simulink model "target"  (R2024b)
settings: Solver=FixedStepDiscrete  StartTime=0.0  StopTime=Inf  FixedStep=0.01  MaxStep=1e-5  RelTol=1e-4  EnableMultiTasking=on
InitFcn:
  | Motor_data_IM_R;
undefined symbols (not defined in the file): DiscIntNeverNeededParam, Down, GPTRIP1SEL, imr_min, j, K_r, K_s, ki, Ki_flux, Ki_w, kp, Kp_flux, Kp_w, lim, p, Tau_r, Ts, TZ1, Up, V_dc, wr_n
libraries: c2802xlib x6, slpidlib x2, c2000lib x1, c280xlib x1
settings Model: ExtModeTrigDuration=8  Creator=dario  LastModifiedBy=dario
settings OptimizationCC: DefaultParameterBehavior=Inlined  DefaultUnderspecifiedDataType=single  EnhancedBackFolding=on  PassReuseOutputArgsAs=Individual arguments  MaxStackSize=1024  OptimizeBlockOrder=speed  DifferentSizesBufferReuse=on  OptimizationCustomize=off  EfficientTunableParamExpr=on
settings DebuggingCC: ParameterTunabilityLossMsg=error
settings HardwareCC: ProdBitPerChar=16  ProdBitPerInt=16  ProdBitPerPointer=32  ProdBitPerSizeT=32  ProdBitPerPtrDiffT=32  ProdLargestAtomicInteger=Integer  ProdLargestAtomicFloat=None  ProdWordSize=16  ProdLongLongMode=on  ProdHWDeviceType=Texas Instruments->C2000  HardwareBoardFeatureSet=SoCBlockset
settings SFSimCC: MATLABDynamicMemAlloc=off
settings RTWCC: Description=Embedded Coder  SystemTargetFile=ert.tlc  HardwareBoard=TI Delfino F28379D LaunchPad  TemplateMakefile=ert_default_tmf  GenerateReport=on  Toolchain=Texas Instruments Code Composer Studio (C2000)  LaunchReport=on  CodeProfilingSaveOptions=MetricsOnly
settings CodeAppCC: ForceParamTrailComments=on  IgnoreCustomStorageClasses=off  OperatorAnnotations=on  SimulinkDataObjDesc=on  SFDataObjDesc=on  InsertBlockDesc=on
settings ERTTargetCC: CodeReplacementLibrary=TI C28x  ExtModeTransport=4  ExtModeStaticAlloc=on  ExtModeAutomaticAllocSize=off  ExtModeStaticAllocSize=10000  ExtModeMexFile=ext_xcp  ExtModeIntrfLevel=Level2 - Open

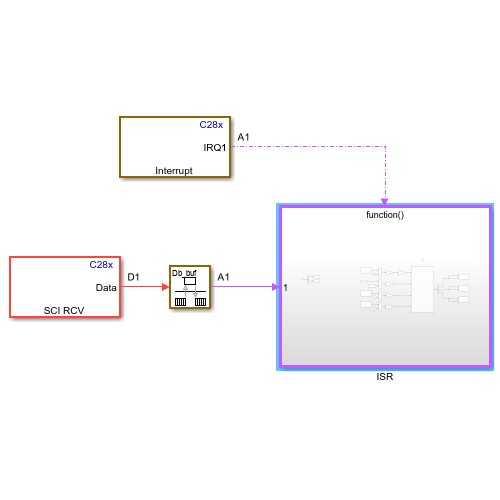
[thumbnail: Simulink's stored preview of the top-level diagram]
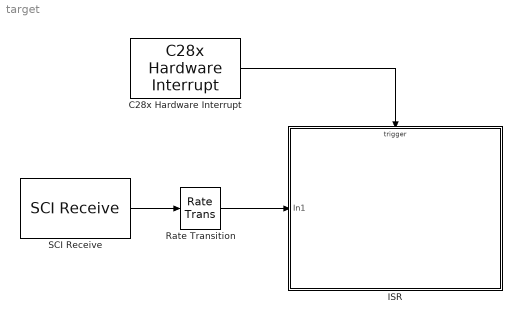
== system target ==
  C28x Hardware Interrupt : c2000lib/Scheduling/C28x Hardware Interrupt  irqnumbers=[1]  pienumbers=[3]  irqpriorities=[30]  irqpreempts=[0]  showinput=off  dspchiptype=C280X
  ISR : Subsystem
  Rate Transition : RateTransition  Deterministic=off
  SCI Receive : c280xlib/SCI Receive  Priority=2  sciModule=A  dataHead='SS'  headerCheckMaxCount=16  dataTail='EE'  dataType=uint16  dataLenOptions=Length via dialog  dataDim=2  maxDataLength=1  initValue=0  errOption=Output the last received value  errValue=0  sampleTime=0.01  blockingMode=off  timeOut=inf  outputStatus=off
      settings: LibrarySourceBlock=c2837xDlib/SCI Receive
  wires:
  C28x Hardware Interrupt/1 -> ISR/Trigger
  Rate Transition/1 -> ISR/1(In1)
  SCI Receive/1 -> Rate Transition/1

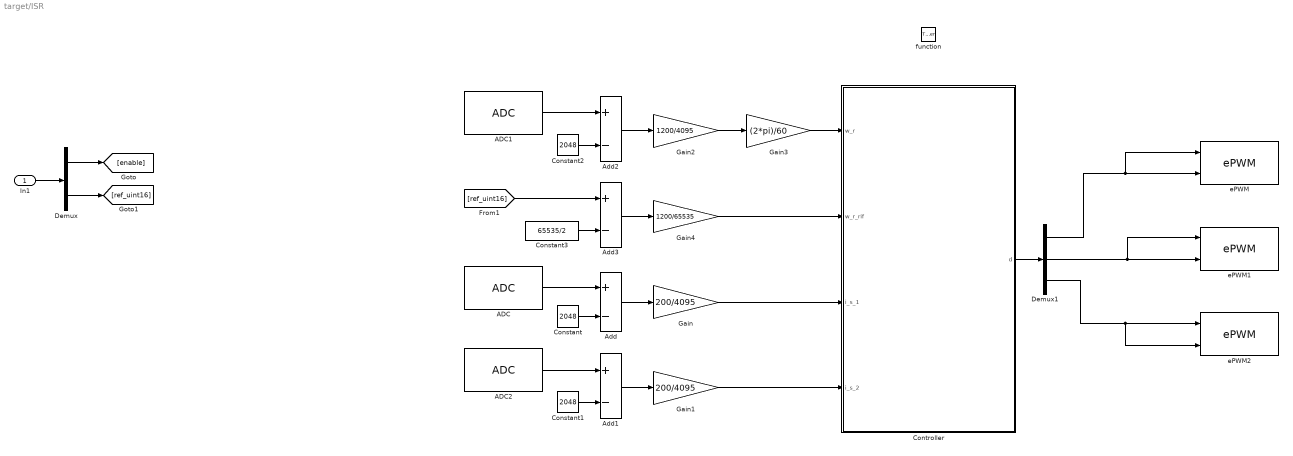
== system target/ISR ==
  In1 : Inport
  function : TriggerPort  TriggerType=function-call  VariantControl=(inherit)
  ADC : c2802xlib/ADC  blkParamProc=C2000_Type4  ADCModule=A  samplingMode=Single sample mode  ADCResolution=12-bit (Single-ended input)  useSOC1=SOC0  useSOC2=SOC0_SOC1  SOCAcquisitionWindow=15  SOCTriggerSource=ePWM1_ADCSOCA  SOCInterruptTrigger=No ADCINT  Ts=-1  dType=uint16  postInterrupt=off  interruptSel=ADCINT1  ADCINTContinuous=on  endma=off  chdma=1  conv1=ADCINA0  conv2=ADCINA0 and ADCINB0  conv1_Type4=ADCIN2  conv2_Type4=ADCIN0 and ADCIN1
      settings: LibrarySourceBlock=c2837xDlib/ADC
  ADC1 : c2802xlib/ADC  blkParamProc=C2000_Type4  ADCModule=C  samplingMode=Single sample mode  ADCResolution=12-bit (Single-ended input)  useSOC1=SOC2  useSOC2=SOC0_SOC1  SOCAcquisitionWindow=15  SOCTriggerSource=ePWM1_ADCSOCA  SOCInterruptTrigger=No ADCINT  Ts=-1  dType=uint16  postInterrupt=on  interruptSel=ADCINT1  ADCINTContinuous=on  endma=off  chdma=1  conv1=ADCINA0  conv2=ADCINA0 and ADCINB0  conv1_Type4=ADCIN2  conv2_Type4=ADCIN0 and ADCIN1
      settings: LibrarySourceBlock=c2837xDlib/ADC
  ADC2 : c2802xlib/ADC  blkParamProc=C2000_Type4  ADCModule=B  samplingMode=Single sample mode  ADCResolution=12-bit (Single-ended input)  useSOC1=SOC1  useSOC2=SOC0_SOC1  SOCAcquisitionWindow=15  SOCTriggerSource=ePWM1_ADCSOCA  SOCInterruptTrigger=No ADCINT  Ts=-1  dType=uint16  postInterrupt=off  interruptSel=ADCINT1  ADCINTContinuous=on  endma=off  chdma=1  conv1=ADCINA0  conv2=ADCINA0 and ADCINB0  conv1_Type4=ADCIN2  conv2_Type4=ADCIN0 and ADCIN1
      settings: LibrarySourceBlock=c2837xDlib/ADC
  Add{,1..3} (4 alike) : Sum  Inputs=+-
  Constant : Constant  Value=2048
  Constant1 : Constant  Value=2048
  Constant2 : Constant  Value=2048
  Constant3 : Constant  Value=65535/2  OutDataTypeStr=single
  Controller : Subsystem
  Demux : Demux  Outputs=2
  Demux1 : Demux  Outputs=3
  Gain : Gain  Gain=200/4095  OutDataTypeStr=single
  Gain1 : Gain  Gain=200/4095  OutDataTypeStr=single
  Gain2 : Gain  Gain=1200/4095  OutDataTypeStr=single
  Gain3 : Gain  Gain=(2*pi)/60  OutDataTypeStr=single
  Gain4 : Gain  Gain=1200/65535  ParamDataTypeStr=single  OutDataTypeStr=single
  ePWM : c2802xlib/ePWM  PwmType=C2000_Type4  useModule=ePWM1  ePWMxLINKTBPRD=Not Linked  periodUnits=Clock cycles  timerSource=Specify via dialog  timerPeriod_clk=5000  timerPeriod_sec=0.0001  tbshadow=Counter equals to zero  countingMode=Up-Down  phaseActiveEnable=Disable  phaseDirection=Count down after sync  phaseActive=0  synchronizationEnable=off  dcaevt1Sync=off  dcbevt1Sync=off  synchronizationOption=Counter equals to zero (CTR=Zero)  dcbevt1SyncOut=off  dcaevt1SyncOut=off  cmpdSyncOut=off  cmpcSyncOut=off  cmpbSyncOut=off  zeroSyncOut=off  swfSyncOut=off  perSynchronizationOption=Counter equals to period (CTR=PRD)  clockPrescale=1  HSclockPrescale=1  enswap=off  ePWMxAStatus=on  ePWMxAactionLogic1=Set  ePWMxAactionLogic2=Clear  ePWMxAactionLogic3=Clear  ePWMxAactionLogic4=Set  ePWMxAactionLogic5=Do nothing  ePWMxAactionLogic6=Do nothing  ePWMxACSFenable=off  ePWMxACSFvalue=Forcing disable  ePWMxASFreload=Zero  ePWMxBStatus=on  ePWMxBactionLogic1=Clear  ePWMxBactionLogic2=Set  ePWMxBactionLogic3=Do nothing  ePWMxBactionLogic4=Do nothing  ePWMxBactionLogic5=Set  ePWMxBactionLogic6=Clear  ePWMxBCSFenable=off  ePWMxBCSFvalue=Forcing disable  ePWMxBSFreload=Zero  ePWNxBOutWay=off  ePWMxLINKCMPA=Not Linked  CMPAUnits=Clock cycles  CMPASource=Input port  CMPAValue_per=50  CMPAValue_clk=32000  enCMPAshadow=Counter equals to zero (CTR=Zero)  ePWMxLINKCMPB=Not Linked  CMPBUnits=Clock cycles  CMPBSource=Input port  CMPBValue_per=50  CMPBValue_clk=32000  enCMPBshadow=Counter equals to zero (CTR=Zero)  ePWMxLINKCMPC=Not Linked  CMPCUnits=Clock cycles  CMPCSource=Specify via dialog  CMPCValue_per=50  CMPCValue_clk=32000  enCMPCshadow=Counter equals to zero (CTR=Zero)  ePWMxLINKCMPD=Not Linked  CMPDUnits=Clock cycles  CMPDSource=Specify via dialog  CMPDValue_per=50  CMPDValue_clk=32000  enCMPDshadow=Counter equals to zero (CTR=Zero)  enableDBePWMxA=off  enableDBePWMxB=off  enhalfcycle=off  DBpolarity=Active high (AH)  DBedgeDelay=Positive  DBSource_ePWMxA=ePWMxA  DBSource_ePWMxB=ePWMxA  DBPeriodUnits=Clock cycles  DBperiodSource=Specify via dialog  REDperiod=0  FEDperiod=0  REDperiod_sec=0  FEDperiod_sec=0  LoadModeDBRED=Immediate without using shadow  LoadModeDBFED=Immediate without using shadow  adcstartModuleA=on  adcrequestEventA=First event  adcstartEventA=Digital Compare Module A Event 1 start of conversion (DCAEVT1.soc)  adcstartEventA_type2=Counter equals to zero (CTR=Zero)  adcstartModuleB=off  adcrequestEventB=First event  adcstartEventB=Counter equals to zero (CTR=Zero)  adcstartEventB_type2=Counter equals to zero (CTR=Zero)  intEn=off  intPrd=First event  intSel=Counter equals to zero (CTR=Zero)  intSel_type2=Counter equals to zero (CTR=Zero)  hrpe=off  enHRPWM=off  HRPWM_LoadMode=Counter equals to period (CTR=PRD)  HRPWM_CTLMode=Duty or Period control mode  HRPWM_EDGMode=Both edge  hrpeb=off  enHRPWMB=off  HRPWM_LoadModeB=Counter equals to zero (CTR=ZERO)  HRPWM_CTLModeB=Duty or Period control mode  HRPWM_EDGModeB=Both edge  enHRDBRED=off  enHRDBFED=off  enSFO=on  enautoconv=on  chopperEnable=off  chopperFrequency=1  chopperFirstwidth=1  chopperDuty=12.5%  tripZonesource=Specify via dialog  tzselOSHT1=off  tzselOSHT2=off  tzselOSHT3=off  tzselOSHT4=off  tzselOSHT5=off  tzselOSHT6=off  tzselOSHDCAEV1=off  tzselOSHDCBEV1=off  tzselCBC1=off  tzselCBC2=off  tzselCBC3=off  tzselCBC4=off  tzselCBC5=off  tzselCBC6=off  tzselCBCDCAEV2=off  tzselCBCDCBEV2=off  enTzOstIntr=off  enTzCbcIntr=off  enTzDCAEVT1Intr=off  enTzDCAEVT2Intr=off  enTzDCBEVT1Intr=off  enTzDCBEVT2Intr=off  tzclrCBCLatch=Counter equals to zero (CTR=Zero)  ePWMxAforced=No action  ePWMxBforced=No action  DCAEVT1forced=No action  DCBEVT1forced=No action  DCAEVT2forced=No action  DCBEVT2forced=No action  dcah=Trip Zone 1 input (TZ1)  dcal=Trip Zone 2 input (TZ2)  dcbh=Trip Zone 1 input (TZ1)  dcbl=Trip Zone 2 input (TZ2)  dcah_type2=GPTRIP1SEL/(TZ1)  dcal_type2=GPTRIP1SEL/(TZ1)  dcbh_type2=GPTRIP1SEL/(TZ1)  dcbl_type2=GPTRIP1SEL/(TZ1)  gendcaevt1=Event disabled  gendcaevt2=Event disabled  gendcbevt1=Event disabled  gendcbevt2=Event disabled  dcaevt1src=DCAEVT1 with sync  dcaevt2src=DCAEVT2 with sync  dcbevt1src=DCBEVT1 with sync  dcbevt2src=DCBEVT2 with sync  pulsesel=Counter equals to zero (CTR=Zero)  blankinv=off  blankoffset=0  blankwidth=0  evsrcsel=Filtered version of DCAEVT1 (DCAEVT1FILT)  encape=off
      settings: LibrarySourceBlock=c2837xDlib/ePWM
  ePWM1 : c2802xlib/ePWM  PwmType=C2000_Type4  useModule=ePWM2  ePWMxLINKTBPRD=Not Linked  periodUnits=Clock cycles  timerSource=Specify via dialog  timerPeriod_clk=5000  timerPeriod_sec=0.0001  tbshadow=Counter equals to zero  countingMode=Up-Down  phaseActiveEnable=Set counter to phase value specified via dialog  phaseDirection=Count up after sync  phaseActive=0  synchronizationEnable=off  dcaevt1Sync=off  dcbevt1Sync=off  synchronizationOption=Counter equals to zero (CTR=Zero)  dcbevt1SyncOut=off  dcaevt1SyncOut=off  cmpdSyncOut=off  cmpcSyncOut=off  cmpbSyncOut=off  zeroSyncOut=off  swfSyncOut=off  perSynchronizationOption=Counter equals to period (CTR=PRD)  clockPrescale=1  HSclockPrescale=1  enswap=off  ePWMxAStatus=on  ePWMxAactionLogic1=Set  ePWMxAactionLogic2=Clear  ePWMxAactionLogic3=Clear  ePWMxAactionLogic4=Set  ePWMxAactionLogic5=Do nothing  ePWMxAactionLogic6=Do nothing  ePWMxACSFenable=off  ePWMxACSFvalue=Forcing disable  ePWMxASFreload=Zero  ePWMxBStatus=on  ePWMxBactionLogic1=Clear  ePWMxBactionLogic2=Set  ePWMxBactionLogic3=Do nothing  ePWMxBactionLogic4=Do nothing  ePWMxBactionLogic5=Set  ePWMxBactionLogic6=Clear  ePWMxBCSFenable=off  ePWMxBCSFvalue=Forcing disable  ePWMxBSFreload=Zero  ePWNxBOutWay=off  ePWMxLINKCMPA=Not Linked  CMPAUnits=Clock cycles  CMPASource=Input port  CMPAValue_per=50  CMPAValue_clk=32000  enCMPAshadow=Counter equals to zero (CTR=Zero)  ePWMxLINKCMPB=Not Linked  CMPBUnits=Clock cycles  CMPBSource=Input port  CMPBValue_per=50  CMPBValue_clk=32000  enCMPBshadow=Counter equals to zero (CTR=Zero)  ePWMxLINKCMPC=Not Linked  CMPCUnits=Clock cycles  CMPCSource=Specify via dialog  CMPCValue_per=50  CMPCValue_clk=32000  enCMPCshadow=Counter equals to zero (CTR=Zero)  ePWMxLINKCMPD=Not Linked  CMPDUnits=Clock cycles  CMPDSource=Specify via dialog  CMPDValue_per=50  CMPDValue_clk=32000  enCMPDshadow=Counter equals to zero (CTR=Zero)  enableDBePWMxA=off  enableDBePWMxB=off  enhalfcycle=off  DBpolarity=Active high (AH)  DBedgeDelay=Positive  DBSource_ePWMxA=ePWMxA  DBSource_ePWMxB=ePWMxA  DBPeriodUnits=Clock cycles  DBperiodSource=Specify via dialog  REDperiod=0  FEDperiod=0  REDperiod_sec=0  FEDperiod_sec=0  LoadModeDBRED=Immediate without using shadow  LoadModeDBFED=Immediate without using shadow  adcstartModuleA=off  adcrequestEventA=First event  adcstartEventA=Digital Compare Module A Event 1 start of conversion (DCAEVT1.soc)  adcstartEventA_type2=Counter equals to zero (CTR=Zero)  adcstartModuleB=off  adcrequestEventB=First event  adcstartEventB=Counter equals to zero (CTR=Zero)  adcstartEventB_type2=Counter equals to zero (CTR=Zero)  intEn=off  intPrd=First event  intSel=Counter equals to zero (CTR=Zero)  intSel_type2=Counter equals to zero (CTR=Zero)  hrpe=off  enHRPWM=off  HRPWM_LoadMode=Counter equals to period (CTR=PRD)  HRPWM_CTLMode=Duty or Period control mode  HRPWM_EDGMode=Both edge  hrpeb=off  enHRPWMB=off  HRPWM_LoadModeB=Counter equals to zero (CTR=ZERO)  HRPWM_CTLModeB=Duty or Period control mode  HRPWM_EDGModeB=Both edge  enHRDBRED=off  enHRDBFED=off  enSFO=on  enautoconv=on  chopperEnable=off  chopperFrequency=1  chopperFirstwidth=1  chopperDuty=12.5%  tripZonesource=Specify via dialog  tzselOSHT1=off  tzselOSHT2=off  tzselOSHT3=off  tzselOSHT4=off  tzselOSHT5=off  tzselOSHT6=off  tzselOSHDCAEV1=off  tzselOSHDCBEV1=off  tzselCBC1=off  tzselCBC2=off  tzselCBC3=off  tzselCBC4=off  tzselCBC5=off  tzselCBC6=off  tzselCBCDCAEV2=off  tzselCBCDCBEV2=off  enTzOstIntr=off  enTzCbcIntr=off  enTzDCAEVT1Intr=off  enTzDCAEVT2Intr=off  enTzDCBEVT1Intr=off  enTzDCBEVT2Intr=off  tzclrCBCLatch=Counter equals to zero (CTR=Zero)  ePWMxAforced=No action  ePWMxBforced=No action  DCAEVT1forced=No action  DCBEVT1forced=No action  DCAEVT2forced=No action  DCBEVT2forced=No action  dcah=Trip Zone 1 input (TZ1)  dcal=Trip Zone 2 input (TZ2)  dcbh=Trip Zone 1 input (TZ1)  dcbl=Trip Zone 2 input (TZ2)  dcah_type2=GPTRIP1SEL/(TZ1)  dcal_type2=GPTRIP1SEL/(TZ1)  dcbh_type2=GPTRIP1SEL/(TZ1)  dcbl_type2=GPTRIP1SEL/(TZ1)  gendcaevt1=Event disabled  gendcaevt2=Event disabled  gendcbevt1=Event disabled  gendcbevt2=Event disabled  dcaevt1src=DCAEVT1 with sync  dcaevt2src=DCAEVT2 with sync  dcbevt1src=DCBEVT1 with sync  dcbevt2src=DCBEVT2 with sync  pulsesel=Counter equals to zero (CTR=Zero)  blankinv=off  blankoffset=0  blankwidth=0  evsrcsel=Filtered version of DCAEVT1 (DCAEVT1FILT)  encape=off
      settings: LibrarySourceBlock=c2837xDlib/ePWM
  ePWM2 : c2802xlib/ePWM  PwmType=C2000_Type4  useModule=ePWM3  ePWMxLINKTBPRD=Not Linked  periodUnits=Clock cycles  timerSource=Specify via dialog  timerPeriod_clk=5000  timerPeriod_sec=0.0001  tbshadow=Counter equals to zero  countingMode=Up-Down  phaseActiveEnable=Set counter to phase value specified via dialog  phaseDirection=Count up after sync  phaseActive=0  synchronizationEnable=off  dcaevt1Sync=off  dcbevt1Sync=off  synchronizationOption=Counter equals to zero (CTR=Zero)  dcbevt1SyncOut=off  dcaevt1SyncOut=off  cmpdSyncOut=off  cmpcSyncOut=off  cmpbSyncOut=off  zeroSyncOut=off  swfSyncOut=off  perSynchronizationOption=Counter equals to period (CTR=PRD)  clockPrescale=1  HSclockPrescale=1  enswap=off  ePWMxAStatus=on  ePWMxAactionLogic1=Set  ePWMxAactionLogic2=Clear  ePWMxAactionLogic3=Clear  ePWMxAactionLogic4=Set  ePWMxAactionLogic5=Do nothing  ePWMxAactionLogic6=Do nothing  ePWMxACSFenable=off  ePWMxACSFvalue=Forcing disable  ePWMxASFreload=Zero  ePWMxBStatus=on  ePWMxBactionLogic1=Clear  ePWMxBactionLogic2=Set  ePWMxBactionLogic3=Do nothing  ePWMxBactionLogic4=Do nothing  ePWMxBactionLogic5=Set  ePWMxBactionLogic6=Clear  ePWMxBCSFenable=off  ePWMxBCSFvalue=Forcing disable  ePWMxBSFreload=Zero  ePWNxBOutWay=off  ePWMxLINKCMPA=Not Linked  CMPAUnits=Clock cycles  CMPASource=Input port  CMPAValue_per=50  CMPAValue_clk=32000  enCMPAshadow=Counter equals to zero (CTR=Zero)  ePWMxLINKCMPB=Not Linked  CMPBUnits=Clock cycles  CMPBSource=Input port  CMPBValue_per=50  CMPBValue_clk=32000  enCMPBshadow=Counter equals to zero (CTR=Zero)  ePWMxLINKCMPC=Not Linked  CMPCUnits=Clock cycles  CMPCSource=Specify via dialog  CMPCValue_per=50  CMPCValue_clk=32000  enCMPCshadow=Counter equals to zero (CTR=Zero)  ePWMxLINKCMPD=Not Linked  CMPDUnits=Clock cycles  CMPDSource=Specify via dialog  CMPDValue_per=50  CMPDValue_clk=32000  enCMPDshadow=Counter equals to zero (CTR=Zero)  enableDBePWMxA=off  enableDBePWMxB=off  enhalfcycle=off  DBpolarity=Active high (AH)  DBedgeDelay=Positive  DBSource_ePWMxA=ePWMxA  DBSource_ePWMxB=ePWMxA  DBPeriodUnits=Clock cycles  DBperiodSource=Specify via dialog  REDperiod=0  FEDperiod=0  REDperiod_sec=0  FEDperiod_sec=0  LoadModeDBRED=Immediate without using shadow  LoadModeDBFED=Immediate without using shadow  adcstartModuleA=off  adcrequestEventA=First event  adcstartEventA=Digital Compare Module A Event 1 start of conversion (DCAEVT1.soc)  adcstartEventA_type2=Counter equals to zero (CTR=Zero)  adcstartModuleB=off  adcrequestEventB=First event  adcstartEventB=Counter equals to zero (CTR=Zero)  adcstartEventB_type2=Counter equals to zero (CTR=Zero)  intEn=off  intPrd=First event  intSel=Counter equals to zero (CTR=Zero)  intSel_type2=Counter equals to zero (CTR=Zero)  hrpe=off  enHRPWM=off  HRPWM_LoadMode=Counter equals to period (CTR=PRD)  HRPWM_CTLMode=Duty or Period control mode  HRPWM_EDGMode=Both edge  hrpeb=off  enHRPWMB=off  HRPWM_LoadModeB=Counter equals to zero (CTR=ZERO)  HRPWM_CTLModeB=Duty or Period control mode  HRPWM_EDGModeB=Both edge  enHRDBRED=off  enHRDBFED=off  enSFO=on  enautoconv=on  chopperEnable=off  chopperFrequency=1  chopperFirstwidth=1  chopperDuty=12.5%  tripZonesource=Specify via dialog  tzselOSHT1=off  tzselOSHT2=off  tzselOSHT3=off  tzselOSHT4=off  tzselOSHT5=off  tzselOSHT6=off  tzselOSHDCAEV1=off  tzselOSHDCBEV1=off  tzselCBC1=off  tzselCBC2=off  tzselCBC3=off  tzselCBC4=off  tzselCBC5=off  tzselCBC6=off  tzselCBCDCAEV2=off  tzselCBCDCBEV2=off  enTzOstIntr=off  enTzCbcIntr=off  enTzDCAEVT1Intr=off  enTzDCAEVT2Intr=off  enTzDCBEVT1Intr=off  enTzDCBEVT2Intr=off  tzclrCBCLatch=Counter equals to zero (CTR=Zero)  ePWMxAforced=No action  ePWMxBforced=No action  DCAEVT1forced=No action  DCBEVT1forced=No action  DCAEVT2forced=No action  DCBEVT2forced=No action  dcah=Trip Zone 1 input (TZ1)  dcal=Trip Zone 2 input (TZ2)  dcbh=Trip Zone 1 input (TZ1)  dcbl=Trip Zone 2 input (TZ2)  dcah_type2=GPTRIP1SEL/(TZ1)  dcal_type2=GPTRIP1SEL/(TZ1)  dcbh_type2=GPTRIP1SEL/(TZ1)  dcbl_type2=GPTRIP1SEL/(TZ1)  gendcaevt1=Event disabled  gendcaevt2=Event disabled  gendcbevt1=Event disabled  gendcbevt2=Event disabled  dcaevt1src=DCAEVT1 with sync  dcaevt2src=DCAEVT2 with sync  dcbevt1src=DCBEVT1 with sync  dcbevt2src=DCBEVT2 with sync  pulsesel=Counter equals to zero (CTR=Zero)  blankinv=off  blankoffset=0  blankwidth=0  evsrcsel=Filtered version of DCAEVT1 (DCAEVT1FILT)  encape=off
      settings: LibrarySourceBlock=c2837xDlib/ePWM
  wires:
  Gain1/1 -> Controller/4(i_s_2)
  ADC/1 -> Add/1
  Add/1 -> Gain/1
  Controller/1(d) -> Demux1/1
  Demux1/1 -> ePWM/1, ePWM/2
  Gain/1 -> Controller/3(i_s_1)
  Demux1/2 -> ePWM1/2, ePWM1/1
  ADC1/1 -> Add2/1
  Add2/1 -> Gain2/1
  Add1/1 -> Gain1/1
  Gain3/1 -> Controller/1(w_r)
  Demux1/3 -> ePWM2/1, ePWM2/2
  Gain2/1 -> Gain3/1
  Constant2/1 -> Add2/2
  Constant/1 -> Add/2
  ADC2/1 -> Add1/1
  Constant1/1 -> Add1/2
  In1/1 -> Demux/1
  Demux/2 -> [ref_uint16]
  Demux/1 -> [enable]
  Constant3/1 -> Add3/2
  [ref_uint16] -> Add3/1
  Add3/1 -> Gain4/1
  Gain4/1 -> Controller/2(w_r_rif)

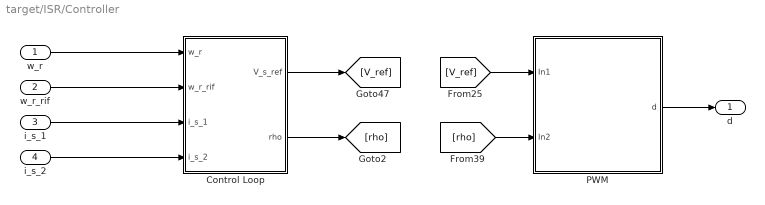
== system target/ISR/Controller ==
  w_r : Inport
  w_r_rif : Inport  Port=2
  i_s_1 : Inport  Port=3
  i_s_2 : Inport  Port=4
  Control Loop : Subsystem
  PWM : Subsystem
  d : Outport
  wires:
  w_r/1 -> Control Loop/1(w_r)
  Control Loop/1(V_s_ref) -> [V_ref]
  w_r_rif/1 -> Control Loop/2(w_r_rif)
  i_s_1/1 -> Control Loop/3(i_s_1)
  i_s_2/1 -> Control Loop/4(i_s_2)
  [V_ref] -> PWM/1(In1)
  PWM/1(d) -> d/1
  [rho] -> PWM/2(In2)
  Control Loop/2(rho) -> [rho]

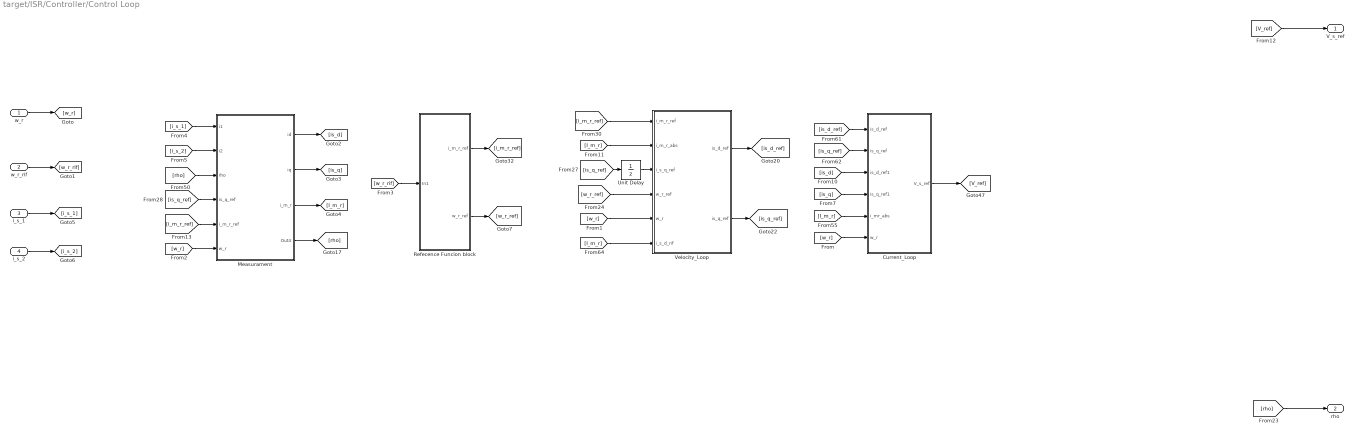
== system target/ISR/Controller/Control Loop ==
  w_r : Inport
  w_r_rif : Inport  Port=2
  i_s_1 : Inport  Port=3
  i_s_2 : Inport  Port=4
  Current_Loop : Subsystem
  Measurament : Subsystem
  Refecence Funcion block : Subsystem
  Unit Delay : UnitDelay  SampleTime=-1  HasFrameUpgradeWarning=on
  Velocity_Loop : Subsystem
  V_s_ref : Outport
  rho : Outport  Port=2
  wires:
  [is_d_ref] -> Current_Loop/1(is_d_ref)
  [is_q] -> Current_Loop/4(is_q_ref1)
  [is_q_ref] -> Unit Delay/1
  [w_r_ref] -> Velocity_Loop/4(w_r_ref)
  [i_m_r_ref] -> Velocity_Loop/1(i_m_r_ref)
  [I_m_r] -> Velocity_Loop/2(i_m_r_abs)
  [is_d] -> Current_Loop/3(is_d_ref1)
  Velocity_Loop/2(is_q_ref) -> [is_q_ref]
  Velocity_Loop/1(is_d_ref) -> [is_d_ref]
  [I_m_r] -> Current_Loop/5(i_mr_abs)
  [is_q_ref] -> Current_Loop/2(is_q_ref)
  Unit Delay/1 -> Velocity_Loop/3(i_s_q_ref)
  [I_m_r] -> Velocity_Loop/6(i_s_d_rif)
  w_r/1 -> [w_r]
  [w_r] -> Velocity_Loop/5(w_r)
  [w_r] -> Current_Loop/6(w_r)
  w_r_rif/1 -> [w_r_rif]
  i_s_1/1 -> [i_s_1]
  i_s_2/1 -> [i_s_2]
  [w_r_rif] -> Refecence Funcion block/1(In1)
  Refecence Funcion block/1(i_m_r_ref) -> [i_m_r_ref]
  [i_s_1] -> Measurament/1(i1)
  [i_s_2] -> Measurament/2(i2)
  [rho] -> Measurament/3(rho)
  [is_q_ref] -> Measurament/4(is_q_ref)
  [i_m_r_ref] -> Measurament/5(i_m_r_ref)
  [w_r] -> Measurament/6(w_r)
  Measurament/1(id) -> [is_d]
  Measurament/2(iq) -> [is_q]
  Measurament/3(i_m_r) -> [I_m_r]
  Measurament/4(Out4) -> [rho]
  Refecence Funcion block/2(w_r_ref) -> [w_r_ref]
  Current_Loop/1(V_s_ref) -> [V_ref]
  [V_ref] -> V_s_ref/1
  [rho] -> rho/1

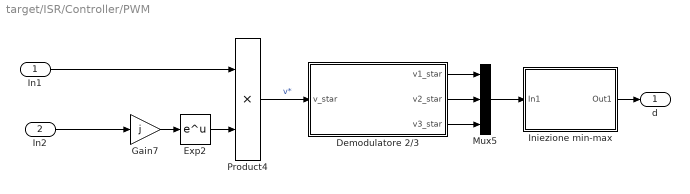
== system target/ISR/Controller/PWM ==
  In1 : Inport
  In2 : Inport  Port=2
  Demodulatore 2/3 : MATLAB Function  TreatAsAtomicUnit=on
  Exp2 : Math  SignedPower=on
  Gain7 : Gain  Gain=j
  Iniezione min-max : Subsystem
  Mux5 : Mux  Inputs=3
  Product4 : Product
  d : Outport
  wires:
  Mux5/1 -> Iniezione min-max/1(In1)
  Demodulatore 2/3/2(v2_star) -> Mux5/2
  Demodulatore 2/3/3(v3_star) -> Mux5/3
  Demodulatore 2/3/1(v1_star) -> Mux5/1
  Iniezione min-max/1(Out1) -> d/1
  Exp2/1 -> Product4/2
  Gain7/1 -> Exp2/1
  In2/1 -> Gain7/1
  Product4/1 -> Demodulatore 2/3/1(v_star)  "v*"
  In1/1 -> Product4/1

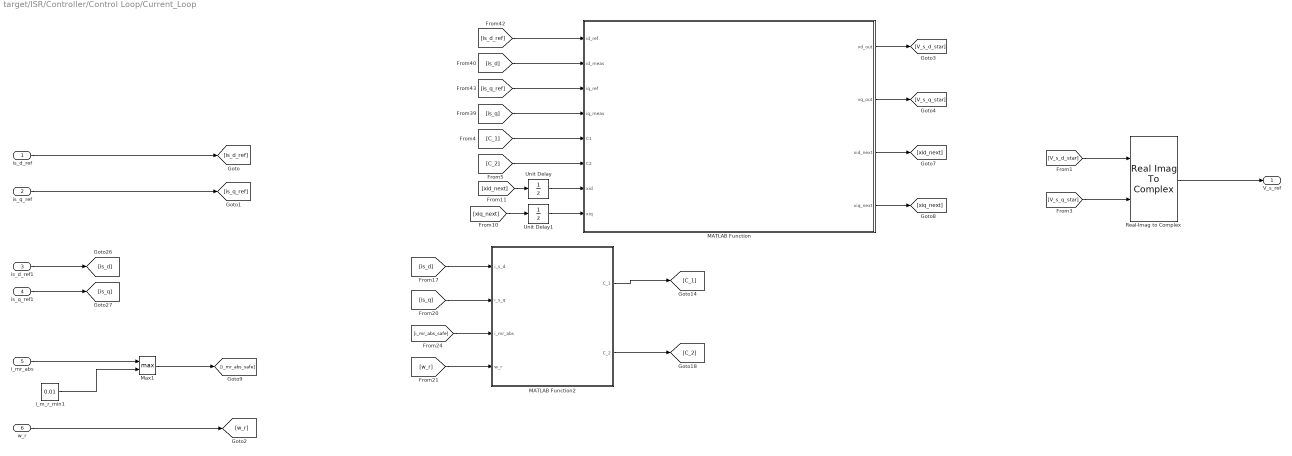
== system target/ISR/Controller/Control Loop/Current_Loop ==
  is_d_ref : Inport
  is_q_ref : Inport  Port=2
  is_d_ref1 : Inport  Port=3
  is_q_ref1 : Inport  Port=4
  i_mr_abs : Inport  Port=5
  w_r : Inport  Port=6
  MATLAB Function : MATLAB Function  TreatAsAtomicUnit=on  mask{Kp_d=kp, Ki_d=ki, Kp_q=kp, Ki_q=ki}
  MATLAB Function2 : MATLAB Function  TreatAsAtomicUnit=on
  Max1 : MinMax  Function=max  Inputs=2
  Real-Imag to Complex : RealImagToComplex
  Unit Delay : UnitDelay  SampleTime=-1  HasFrameUpgradeWarning=on
  Unit Delay1 : UnitDelay  SampleTime=-1  HasFrameUpgradeWarning=on
  i_m_r_min1 : Constant  Value=0.01  OutDataTypeStr=single
  V_s_ref : Outport
  wires:
  is_q_ref1/1 -> [is_q]
  [w_r] -> MATLAB Function2/4(w_r)
  [is_q] -> MATLAB Function2/2(i_s_q)
  [is_d] -> MATLAB Function2/1(i_s_d)
  [i_mr_abs_safe] -> MATLAB Function2/3(i_mr_abs)
  Max1/1 -> [i_mr_abs_safe]
  i_m_r_min1/1 -> Max1/2
  MATLAB Function2/2(C_2) -> [C_2]
  is_d_ref1/1 -> [is_d]
  MATLAB Function2/1(C_1) -> [C_1]
  i_mr_abs/1 -> Max1/1
  is_d_ref/1 -> [is_d_ref]
  is_q_ref/1 -> [is_q_ref]
  w_r/1 -> [w_r]
  Real-Imag to Complex/1 -> V_s_ref/1
  [V_s_d_star] -> Real-Imag to Complex/1
  [V_s_q_star] -> Real-Imag to Complex/2
  [is_d_ref] -> MATLAB Function/1(id_ref)
  [is_d] -> MATLAB Function/2(id_meas)
  [is_q_ref] -> MATLAB Function/3(iq_ref)
  [is_q] -> MATLAB Function/4(iq_meas)
  [C_1] -> MATLAB Function/5(C1)
  [C_2] -> MATLAB Function/6(C2)
  MATLAB Function/1(vd_out) -> [V_s_d_star]
  MATLAB Function/2(vq_out) -> [V_s_q_star]
  MATLAB Function/3(xid_next) -> [xid_next]
  MATLAB Function/4(xiq_next) -> [xiq_next]
  [xid_next] -> Unit Delay/1
  Unit Delay/1 -> MATLAB Function/7(xid)
  [xiq_next] -> Unit Delay1/1
  Unit Delay1/1 -> MATLAB Function/8(xiq)

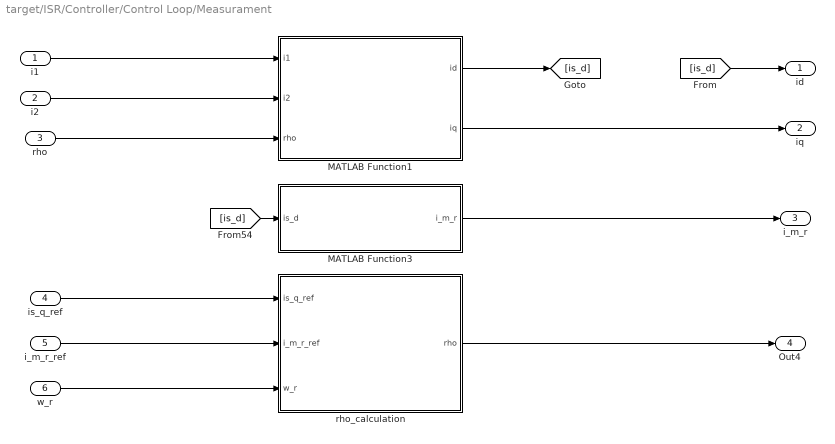
== system target/ISR/Controller/Control Loop/Measurament ==
  i1 : Inport
  i2 : Inport  Port=2
  rho : Inport  Port=3
  is_q_ref : Inport  Port=4
  i_m_r_ref : Inport  Port=5
  w_r : Inport  Port=6
  MATLAB Function1 : MATLAB Function  TreatAsAtomicUnit=on
  MATLAB Function3 : MATLAB Function  TreatAsAtomicUnit=on
  rho_calculation : Subsystem
  id : Outport
  iq : Outport  Port=2
  i_m_r : Outport  Port=3
  Out4 : Outport  Port=4
  wires:
  MATLAB Function3/1(i_m_r) -> i_m_r/1
  i2/1 -> MATLAB Function1/2(i2)
  [is_d] -> MATLAB Function3/1(is_d)
  i1/1 -> MATLAB Function1/1(i1)
  w_r/1 -> rho_calculation/3(w_r)
  MATLAB Function1/2(iq) -> iq/1
  MATLAB Function1/1(id) -> [is_d]
  i_m_r_ref/1 -> rho_calculation/2(i_m_r_ref)
  rho/1 -> MATLAB Function1/3(rho)
  rho_calculation/1(rho) -> Out4/1
  is_q_ref/1 -> rho_calculation/1(is_q_ref)
  [is_d] -> id/1

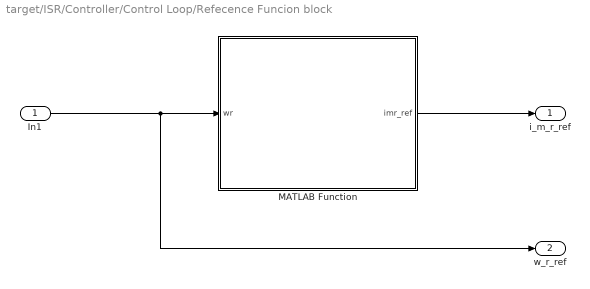
== system target/ISR/Controller/Control Loop/Refecence Funcion block ==
  In1 : Inport
  MATLAB Function : MATLAB Function  TreatAsAtomicUnit=on
  i_m_r_ref : Outport
  w_r_ref : Outport  Port=2
  wires:
  MATLAB Function/1(imr_ref) -> i_m_r_ref/1
  In1/1 -> w_r_ref/1, MATLAB Function/1(wr)

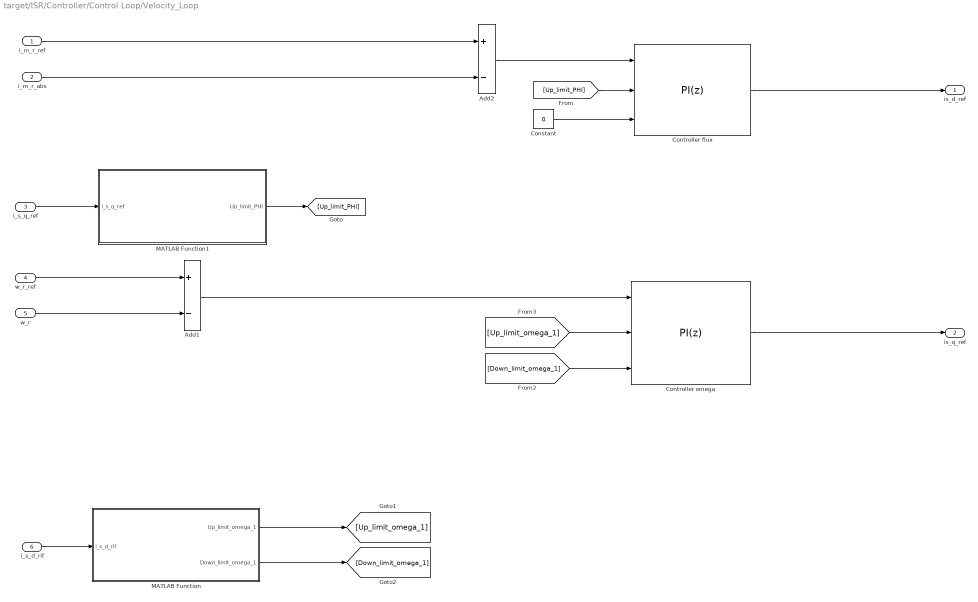
== system target/ISR/Controller/Control Loop/Velocity_Loop ==
  i_m_r_ref : Inport
  i_m_r_abs : Inport  Port=2
  i_s_q_ref : Inport  Port=3
  w_r_ref : Inport  Port=4
  w_r : Inport  Port=5
  i_s_d_rif : Inport  Port=6
  Add1 : Sum  Inputs=+-
  Add2 : Sum  Inputs=+-
  Constant : Constant  Value=0  OutDataTypeStr=single
  Controller flux : slpidlib/PID Controller  Controller=PI  Form=Parallel  TimeDomain=Discrete-time  UseExternalTs=off  SampleTime=-1  IntegratorMethod=Trapezoidal  FilterMethod=Forward Euler  ControllerParametersSource=internal  P=1*Kp_flux  I=1*Ki_flux  UseKiTs=off  D=0  UseExternalDerivativeSource=off  N=100  UseFilter=on  TunerSelectOption=Transfer Function Based (PID Tuner App)  InitialConditionSource=internal  InitialConditionForIntegrator=0  InitialConditionForFilter=0  DifferentiatorICPrevScaledInput=0  ExternalReset=none  TrackingMode=off  Kt=1  LimitOutput=on  SatLimitsSource=external  UpperSaturationLimit=inf  LowerSaturationLimit=-inf  LinearizeAsGain=on  AntiWindupMode=clamping  Kb=1  LimitIntegrator=off  UpperIntegratorSaturationLimit=Up_limit_PHI  LowerIntegratorSaturationLimit=0  POutMin=[]  POutMax=[]  IOutMin=[]  IOutMax=[]  DOutMin=[]  DOutMax=[]  NOutMin=[]  NOutMax=[]  SumOutMin=[]  SumOutMax=[]  SaturationOutMin=[]  SaturationOutMax=[]  PParamMin=[]  PParamMax=[]  IParamMin=[]  IParamMax=[]  DParamMin=[]  DParamMax=[]  NParamMin=[]  NParamMax=[]  KbParamMin=[]  KbParamMax=[]  KtParamMin=[]  KtParamMax=[]  KbOutMin=[]  KbOutMax=[]  KtOutMin=[]  KtOutMax=[]  IntegratorOutMin=[]  IntegratorOutMax=[]  FilterOutMin=[]  FilterOutMax=[]  SumI1OutMin=[]  SumI1OutMax=[]  SumI2OutMin=[]  SumI2OutMax=[]  SumI3OutMin=[]  SumI3OutMax=[]  SumI4OutMin=[]  SumI4OutMax=[]  SumDOutMin=[]  SumDOutMax=[]  DifferentiatorOutMin=[]  DifferentiatorOutMax=[]  FilterDiffOutCoefMin=[]  FilterDiffOutCoefMax=[]  ReciprocalOutMin=[]  ReciprocalOutMax=[]  SumDenOutMin=[]  SumDenOutMax=[]  SumNumOutMin=[]  SumNumOutMax=[]  DivideOutMin=[]  DivideOutMax=[]  UdiffTsProdOutMin=[]  UdiffTsProdOutMax=[]  NTsProdOutMin=[]  NTsProdOutMax=[]  UintegralTsProdOutMin=[]  UintegralTsProdOutMax=[]  UngainTsProdOutMin=[]  UngainTsProdOutMax=[]  ClampingZeroOutDataTypeStr=Inherit: Inherit via back propagation  ClampingZeroOutMin=[]  ClampingZeroOutMax=[]  FilterDenConstantOutDataTypeStr=Inherit: Inherit via back propagation  FilterDenConstantOutMin=[]  FilterDenConstantOutMax=[]  PCopyOutDataTypeStr=Inherit: Inherit via back propagation  PCopyOutMin=[]  PCopyOutMax=[]  NCopyOutDataTypeStr=Inherit: Inherit via back propagation  NCopyOutMin=[]  NCopyOutMax=[]  IntegratorContinuousStateAttributes=''  IntegratorStateMustResolveToSignalObject=off  IntegratorRTWStateStorageClass=Auto  FilterContinuousStateAttributes=''  FilterStateMustResolveToSignalObject=off  FilterRTWStateStorageClass=Auto  ParallelPVariant=InternalParameters  IdealPVariant=Disabled  IVariant=InternalParameters  DVariant=Disabled  IntegratorVariant=Discrete  SatVariant=External  AWVariant=DiscClampingParallel  PCopyVariant=Disabled  TRVariant=Disabled  FdbkBlocksVariant=Feedback  IdealPFdbkVariant=Passthrough  SatFdbkVariant=Passthrough  DerivativeFilterVariant=Disabled  NVariant=Disabled  NCopyVariant=Disabled_SignalSpec  FilterICVariant=Disabled  IntegratorICVariant=InternalICs  ExternalResetVariant=Disabled  TRSumVariant=Passthrough  SumFdbkVariant=Enabled  SumVariant=Sum_PI  TsampFilterVariant=InternalTs  TsampNgainVariant=Passthrough  TsampIntegralVariant=Disabled_SignalSpec  ExternalSaturationOutDataTypeStr=Inherit: Same as second input  DerivativeSourceVariant=Disabled  PreIntVariant=InternalPreInt
  Controller omega : slpidlib/PID Controller  Controller=PI  Form=Parallel  TimeDomain=Discrete-time  UseExternalTs=off  SampleTime=-1  IntegratorMethod=Trapezoidal  FilterMethod=Forward Euler  ControllerParametersSource=internal  P=1*Kp_w  I=1*Ki_w  UseKiTs=off  D=0  UseExternalDerivativeSource=off  N=100  UseFilter=on  TunerSelectOption=Transfer Function Based (PID Tuner App)  InitialConditionSource=internal  InitialConditionForIntegrator=0  InitialConditionForFilter=0  DifferentiatorICPrevScaledInput=0  ExternalReset=none  TrackingMode=off  Kt=1  LimitOutput=on  SatLimitsSource=external  UpperSaturationLimit=inf  LowerSaturationLimit=-inf  LinearizeAsGain=on  AntiWindupMode=clamping  Kb=1  LimitIntegrator=off  UpperIntegratorSaturationLimit=Up_limit_PHI  LowerIntegratorSaturationLimit=0  POutMin=[]  POutMax=[]  IOutMin=[]  IOutMax=[]  DOutMin=[]  DOutMax=[]  NOutMin=[]  NOutMax=[]  SumOutMin=[]  SumOutMax=[]  SaturationOutMin=[]  SaturationOutMax=[]  PParamMin=[]  PParamMax=[]  IParamMin=[]  IParamMax=[]  DParamMin=[]  DParamMax=[]  NParamMin=[]  NParamMax=[]  KbParamMin=[]  KbParamMax=[]  KtParamMin=[]  KtParamMax=[]  KbOutMin=[]  KbOutMax=[]  KtOutMin=[]  KtOutMax=[]  IntegratorOutMin=[]  IntegratorOutMax=[]  FilterOutMin=[]  FilterOutMax=[]  SumI1OutMin=[]  SumI1OutMax=[]  SumI2OutMin=[]  SumI2OutMax=[]  SumI3OutMin=[]  SumI3OutMax=[]  SumI4OutMin=[]  SumI4OutMax=[]  SumDOutMin=[]  SumDOutMax=[]  DifferentiatorOutMin=[]  DifferentiatorOutMax=[]  FilterDiffOutCoefMin=[]  FilterDiffOutCoefMax=[]  ReciprocalOutMin=[]  ReciprocalOutMax=[]  SumDenOutMin=[]  SumDenOutMax=[]  SumNumOutMin=[]  SumNumOutMax=[]  DivideOutMin=[]  DivideOutMax=[]  UdiffTsProdOutMin=[]  UdiffTsProdOutMax=[]  NTsProdOutMin=[]  NTsProdOutMax=[]  UintegralTsProdOutMin=[]  UintegralTsProdOutMax=[]  UngainTsProdOutMin=[]  UngainTsProdOutMax=[]  ClampingZeroOutDataTypeStr=Inherit: Inherit via back propagation  ClampingZeroOutMin=[]  ClampingZeroOutMax=[]  FilterDenConstantOutDataTypeStr=Inherit: Inherit via back propagation  FilterDenConstantOutMin=[]  FilterDenConstantOutMax=[]  PCopyOutDataTypeStr=Inherit: Inherit via back propagation  PCopyOutMin=[]  PCopyOutMax=[]  NCopyOutDataTypeStr=Inherit: Inherit via back propagation  NCopyOutMin=[]  NCopyOutMax=[]  IntegratorContinuousStateAttributes=''  IntegratorStateMustResolveToSignalObject=off  IntegratorRTWStateStorageClass=Auto  FilterContinuousStateAttributes=''  FilterStateMustResolveToSignalObject=off  FilterRTWStateStorageClass=Auto  ParallelPVariant=InternalParameters  IdealPVariant=Disabled  IVariant=InternalParameters  DVariant=Disabled  IntegratorVariant=Discrete  SatVariant=External  AWVariant=DiscClampingParallel  PCopyVariant=Disabled  TRVariant=Disabled  FdbkBlocksVariant=Feedback  IdealPFdbkVariant=Passthrough  SatFdbkVariant=Passthrough  DerivativeFilterVariant=Disabled  NVariant=Disabled  NCopyVariant=Disabled_SignalSpec  FilterICVariant=Disabled  IntegratorICVariant=InternalICs  ExternalResetVariant=Disabled  TRSumVariant=Passthrough  SumFdbkVariant=Enabled  SumVariant=Sum_PI  TsampFilterVariant=InternalTs  TsampNgainVariant=Passthrough  TsampIntegralVariant=Disabled_SignalSpec  ExternalSaturationOutDataTypeStr=Inherit: Same as second input  DerivativeSourceVariant=Disabled  PreIntVariant=InternalPreInt
  MATLAB Function : MATLAB Function  TreatAsAtomicUnit=on
  MATLAB Function1 : MATLAB Function  TreatAsAtomicUnit=on
  is_d_ref : Outport
  is_q_ref : Outport  Port=2
  wires:
  i_m_r_ref/1 -> Add2/1
  w_r/1 -> Add1/2
  i_m_r_abs/1 -> Add2/2
  Add2/1 -> Controller flux/1
  Add1/1 -> Controller omega/1
  w_r_ref/1 -> Add1/1
  Controller omega/1 -> is_q_ref/1
  Controller flux/1 -> is_d_ref/1
  Constant/1 -> Controller flux/3
  [Up_limit_PHI] -> Controller flux/2
  [Up_limit_omega_1] -> Controller omega/2
  [Down_limit_omega_1] -> Controller omega/3
  i_s_d_rif/1 -> MATLAB Function/1(i_s_d_rif)
  MATLAB Function/1(Up_limit_omega_1) -> [Up_limit_omega_1]
  MATLAB Function/2(Down_limit_omega_1) -> [Down_limit_omega_1]
  i_s_q_ref/1 -> MATLAB Function1/1(i_s_q_ref)
  MATLAB Function1/1(Up_limit_PHI) -> [Up_limit_PHI]

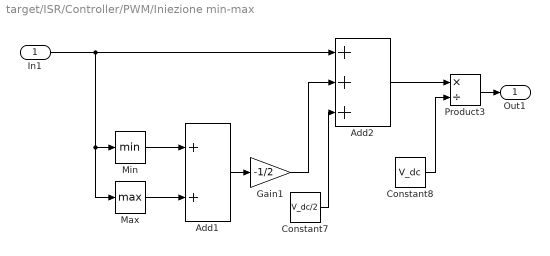
== system target/ISR/Controller/PWM/Iniezione min-max ==
  In1 : Inport
  Add1 : Sum
  Add2 : Sum  Inputs=+++
  Constant7 : Constant  Value=V_dc/2
  Constant8 : Constant  Value=V_dc
  Gain1 : Gain  Gain=-1/2
  Max : MinMax  Function=max
  Min : MinMax
  Product3 : Product  Inputs=*/
  Out1 : Outport
  wires:
  Max/1 -> Add1/2
  Constant7/1 -> Add2/3
  Constant8/1 -> Product3/2
  Min/1 -> Add1/1
  In1/1 -> Max/1, Min/1, Add2/1
  Add1/1 -> Gain1/1
  Gain1/1 -> Add2/2
  Add2/1 -> Product3/1
  Product3/1 -> Out1/1

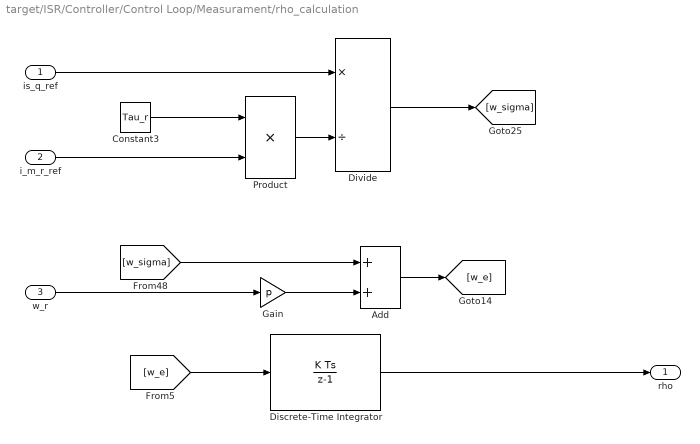
== system target/ISR/Controller/Control Loop/Measurament/rho_calculation ==
  is_q_ref : Inport
  i_m_r_ref : Inport  Port=2
  w_r : Inport  Port=3
  Add : Sum
  Constant3 : Constant  Value=Tau_r
  Discrete-Time Integrator : DiscreteIntegrator  SampleTime=-1  OutDataTypeStr=single  ICPrevOutput=DiscIntNeverNeededParam  ICPrevScaledInput=DiscIntNeverNeededParam
  Divide : Product  Inputs=*/
  Gain : Gain  Gain=p
  Product : Product
  rho : Outport
  wires:
  Gain/1 -> Add/2
  Product/1 -> Divide/2
  Divide/1 -> [w_sigma]
  Constant3/1 -> Product/1
  [w_sigma] -> Add/1
  Add/1 -> [w_e]
  i_m_r_ref/1 -> Product/2
  [w_e] -> Discrete-Time Integrator/1
  w_r/1 -> Gain/1
  is_q_ref/1 -> Divide/1
  Discrete-Time Integrator/1 -> rho/1

== matlab function target/ISR/Controller/PWM/Demodulatore 2//3 ==
  settings: updateMethod=DISCRETE
  data: v_star input; v1_star output; v2_star output; v3_star output
function [v1_star, v2_star, v3_star] = demodulation(v_star)
v1_star=real(v_star);
v2_star=-1/2*real(v_star)+sqrt(3)/2*imag(v_star);
v3_star=-1/2*real(v_star)-sqrt(3)/2*imag(v_star);

== matlab function target/ISR/Controller/Control Loop/Current_Loop/MATLAB Function ==
  data: id_ref input single; vd_out output single; id_meas input single; iq_ref input single; iq_meas input single; C1 input single; C2 input single; xid input single; xiq input single; vq_out output single; xid_next output single; xiq_next output single; Ki_d parameter double; lim parameter single; Ts parameter single; Kp_d parameter single; Ki_q parameter single; Kp_q parameter single
function [vd_out, vq_out, xid_next, xiq_next] = foc_vdq_pi_aw_min( ...
    id_ref, id_meas, iq_ref, iq_meas, ...
    C1, C2, xid, xiq, Ki_d, lim, Ts, ...
Kp_d, Ki_q, ...
Kp_q)
%#codegen
% MINIMO: PI(d,q) + C1/C2 + saturazione vettoriale + anti-windup back-calculation
% Stati integratori gestiti esternamente (Unit Delay / Discrete-Time Integrator)

% --- Anti-windup gain (regola pratica) ---
epsKp = single(1e-12);
Kaw_d = Ki_d / max(abs(Kp_d), epsKp);
Kaw_q = Ki_q / max(abs(Kp_q), epsKp);

% --- Errori ---
ed = id_ref - id_meas;
eq = iq_ref - iq_meas;

% --- PI + compensazioni (non saturato) ---
vd_unsat = (Kp_d * ed + xid) + C1;
vq_unsat = (Kp_q * eq + xiq) + C2;

% --- Saturazione vettoriale ---
Vmag  = sqrt(vd_unsat*vd_unsat + vq_unsat*vq_unsat);
Vsafe = max(Vmag, 1e-12);

k = lim / Vsafe;
if k > single(1)
    k = single(1);
elseif k < single(0)
    k = single(0);
end

vd_out = vd_unsat * k;
vq_out = vq_unsat * k;

% --- Anti-windup back-calculation ---
awd = vd_out - vd_unsat;
awq = vq_out - vq_unsat;

% --- Update integratori ---
xid_next = xid + Ts*(Ki_d*ed + Kaw_d*awd);
xiq_next = xiq + Ts*(Ki_q*eq + Kaw_q*awq);

end

== matlab function target/ISR/Controller/Control Loop/Measurament/MATLAB Function1 ==
  data: i1 input single; id output single; i2 input single; rho input single; iq output single
function [id, iq] = meas_fast(i1, i2, rho)
%#codegen
i1  = single(i1);
i2  = single(i2);
rho = single(rho);

inv_sqrt3 = single(0.5773502691896258); % 1/sqrt(3)

ialpha = i1;
ibeta  = inv_sqrt3 * (i1 + single(2)*i2);

c = cos(rho);
s = sin(rho);

id = ialpha*c + ibeta*s;
iq = ibeta*c - ialpha*s;
end

== matlab function target/ISR/Controller/Control Loop/Measurament/MATLAB Function3 ==
  data: is_d input; i_m_r output; Ts parameter; Tau_r parameter
function i_m_r = i_m_r_calculation(is_d, Ts, Tau_r)
%#codegen

persistent i_m_z
if isempty(i_m_z)
    i_m_z = single(0);
end

Tau_min = single(1e-6);
Tr = max(Tau_r, Tau_min);

i_m_z = i_m_z + (Ts/Tr) * (is_d - i_m_z);
i_m_r = i_m_z;
end

== matlab function target/ISR/Controller/Control Loop/Velocity_Loop/MATLAB Function ==
  settings: updateMethod=DISCRETE
  data: i_s_d_rif input single; Up_limit_omega_1 output single; Is_adc parameter single; Down_limit_omega_1 output single
function [Up_limit_omega_1,Down_limit_omega_1]   = sqrt_max_diff(i_s_d_rif, Is_adc)

v = Is_adc*Is_adc - i_s_d_rif*i_s_d_rif;   % i_s_d_rif^2 - I_s_max^2
v = max(v, single(0));

Up_limit_omega_1 = sqrt(v);
Down_limit_omega_1=-Up_limit_omega_1;
end

== matlab function target/ISR/Controller/Control Loop/Current_Loop/MATLAB Function2 ==
  data: i_s_d input single; C_1 output single; i_s_q input single; i_mr_abs input single; w_r input single; C_2 output single; p parameter single; Tau_r parameter single; K_s parameter single; K_r parameter single
function [C_1, C_2] = fcn(i_s_d, i_s_q, i_mr_abs, w_r, p, Tau_r, K_s, K_r)
%#codegen

    critic_elem_1 = i_s_q / (Tau_r * i_mr_abs);
    critic_elem_2  = p * w_r + critic_elem_1;

    %--- Compensazioni (come schema AEAR)
    C_1 = (K_r/Tau_r) * (i_s_d - i_mr_abs) - K_s * i_s_q * critic_elem_2;
    C_2 = (K_s * i_s_d + K_r * i_mr_abs) * critic_elem_2;

end

== matlab function target/ISR/Controller/Control Loop/Refecence Funcion block/MATLAB Function ==
  data: wr input single; imr_ref output single; wr_n parameter single; imr_min parameter single
function imr_ref = imr_ref_from_wr(wr, wr_n, imr_min)
% wr     : velocità rotorica [rad/s]
% wr_n   : velocità base [rad/s] (deve essere >0)
% imr_ref_peak : corrente magnetizzante nominale (picco o dq coerente)
% imr_min: minimo ammesso

wr_abs  = abs(wr);
ref=single(35);
% Guardia su wr_n (evita wr_n=0/negativo/non inizializzato)
% if ~(isfinite(wr_n_abs) && wr_n_abs > 0)
%     imr_ref = imr_ref_peak;   % fallback: flusso nominale
%     return;
% end

if wr_abs <= wr_n
   imr_ref = ref;
else
   imr_ref = ref * (wr_n / wr_abs); % iperbolica
end

% % Guardia su avviamento / velocità ~0
% w_eps = 1e-3; % [rad/s] soglia (puoi alzare a 1e-2 se vuoi)
% if wr_abs < w_eps
%     imr_ref = single(25);
% else
%     if wr_abs <= wr_n_abs
%         imr_ref = single(25);
%     else
%         imr_ref = imr_ref_peak * (wr_n_abs / wr_abs); % iperbolica
%     end
% end

% % saturazione finale
imr_ref = max(imr_min, imr_ref);
end

== matlab function target/ISR/Controller/Control Loop/Velocity_Loop/MATLAB Function1 ==
  settings: updateMethod=DISCRETE
  data: i_s_q_ref input single; Up_limit_PHI output single; Is_adc parameter
function Up_limit_PHI    = sqrt_max_diff(i_s_q_ref, Is_adc)

v = Is_adc*Is_adc - i_s_q_ref*i_s_q_ref;   % i_s_q_ref^2 - I_base_max^2
v = max(v, single(0));

Up_limit_PHI = sqrt(v);

end
